simulink model "Solar_Vector_Control"  (R2024b)
settings: Solver=ode23t  StartTime=0.0  StopTime=2.5  RelTol=1e-3
libraries: spsCurrentMeasurementLib x6, spsVoltageMeasurementLib x4, spsSeriesRLCBranchLib x3, simulink x2, slpidlib x2, spsDiodeLib x1, spsIGBTLib x1, spsAsynchronousMachineSIUnitsLib x1, spsPVArrayLib x1, spsUniversalBridgeLib x1, spspowerguiLib x1
settings Model: Creator=ASUS  LastModifiedBy=ASUS
settings SolverCC: ZeroCrossControl=DisableAll

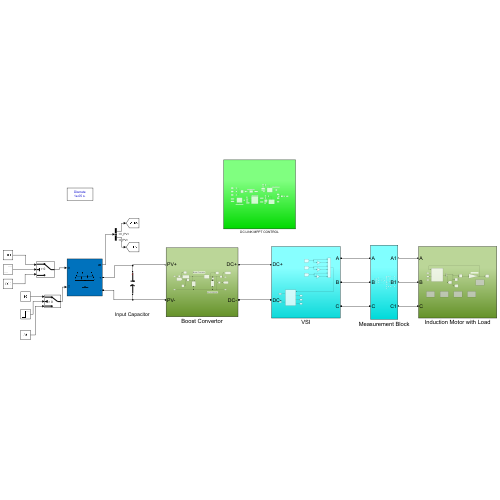
[thumbnail: Simulink's stored preview of the top-level diagram]
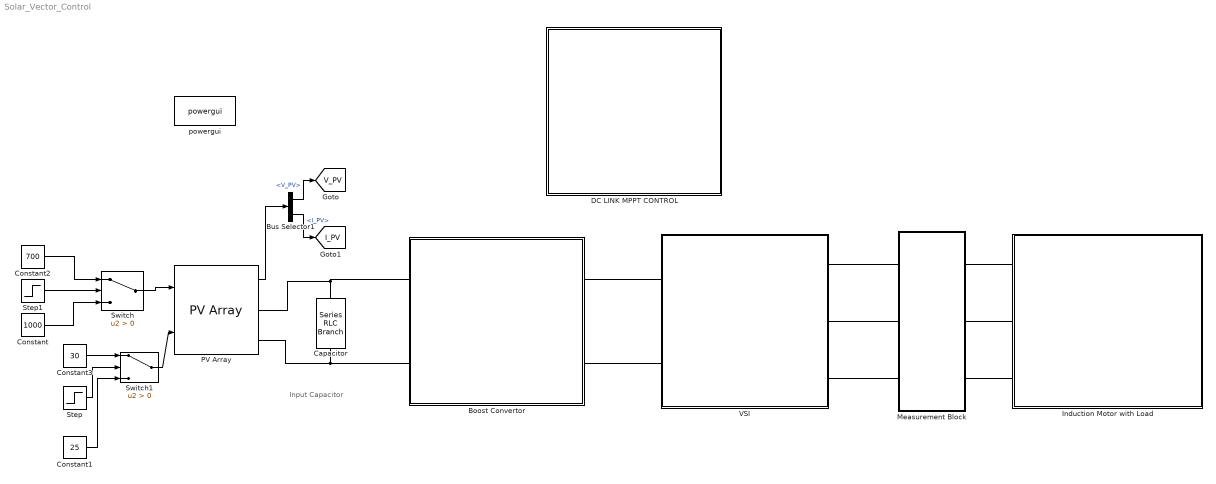
== system Solar_Vector_Control ==
  note: Input Capacitor
  Boost Convertor : Subsystem
  Bus Selector1 : BusSelector  OutputSignals=V_PV,I_PV
  Capacitor : spsSeriesRLCBranchLib/Series RLC Branch  LConnTagsString=__new0  RConnTagsString=__new0  BranchType=C  Resistance=1  Inductance=1e-3  SetiL0=off  InitialCurrent=0  Capacitance=100e-6  Setx0=off  InitialVoltage=0  Measurements=None
  Constant : Constant  Value=1000
  Constant1 : Constant  Value=25
  Constant2 : Constant  Value=700
  Constant3 : Constant  Value=30
  DC LINK MPPT CONTROL : Subsystem
  Induction Motor with Load : Subsystem
  Measurement Block : Subsystem
  PV Array : spsPVArrayLib/PV Array  Npar=2  Nser=12  PlotType=array @ 1000 W/m2 & specified temperatures  S_vec="[ 1000  500  100 ]"  Temp_C_vec="[ 45 25  ]"  ModuleName=User-defined  PlotWhenSelected=off  Pm=213.15  Ncell=60  Voc=36.3  Isc=7.84  Vm=29  Im=7.35  beta_Voc_pc=-0.36099  alpha_Isc_pc=0.102  beta_Voc=-0.13104  alpha_Isc=0.0079968  IL=7.8654  I0=2.9273e-10  nI=0.98119  Rsh=313.0553  Rs=0.39381  RobustModel=off  RobustCellTemperature=313.3991  BAL=on  Tc=1e-6  Tfilter=5e-5
  Step : Step  Time=5  SampleTime=0
  Step1 : Step  Time=3  SampleTime=0
  Switch : Switch  Criteria=u2 > Threshold  SaturateOnIntegerOverflow=off  InputSameDT=off
  Switch1 : Switch  Criteria=u2 > Threshold  SaturateOnIntegerOverflow=off  InputSameDT=off
  VSI : Subsystem
  powergui : spspowerguiLib/powergui  Priority=1  SimulationMode=Discrete  SampleTime=10e-6  frequency=60  Iterations=50  frequencyindice=0  Pbase=100e6  ErrMax=1e-4  UnitsV=kV  UnitsW=MW  buscounter=0  FunctionMessages=off  echomessages=off  EnableUseOfTLC=off  CurrentSourceSwitches=off  DisableSnubberDevices=off  DisableRonSwitches=off  DisableVfSwitches=off  DisplayEquations=off  AutomaticDiscreteSolvers=off  SolverType=Tustin/Backward Euler (TBE)  Interpol=off  ExternalGateDelay=off  methode=off  Ts=100  x0status=blocks  SPID=on  SwTol=0  HookPort=off  NonlinearTolerance=1e-4  nMaxIteration=100  ContinueOnMaxIteration=off  RestoreLinks=warning  ResistiveCurrentMeasurement=off  Frange=[0:2:500]  Ylog=off  Xlog=on  ShowGrid=off  save=off  variable=ZData  structure=0  ZoomFFT=off  StartTime=0.0  cycles=1  DisplayStyle=1  fundamental=60  FreqAxis=off  MaxFrequency=1000  frequencyindicesteady=1  RmsSteady=1  display=off
  tag scope: I_PV=global, V_PV=global
  wires:
  Switch/1 -> PV Array/1
  PV Array/1 -> Bus Selector1/1
  Bus Selector1/1 -> [V_PV]  "<V_PV>"
  Bus Selector1/2 -> [I_PV]  "<I_PV>"
  Constant/1 -> Switch/3
  Constant2/1 -> Switch/1
  Switch1/1 -> PV Array/2
  Constant1/1 -> Switch1/3
  Constant3/1 -> Switch1/1
  Step/1 -> Switch1/2
  Step1/1 -> Switch/2
  connections:
  PV Array/RConn1 -- Boost Convertor/LConn1 -- Capacitor/LConn1
  Capacitor/RConn1 -- PV Array/RConn2 -- Boost Convertor/LConn2
  Measurement Block/LConn1 -- VSI/LConn1
  VSI/LConn2 -- Measurement Block/LConn2
  Measurement Block/RConn2 -- Induction Motor with Load/LConn2
  Measurement Block/RConn1 -- Induction Motor with Load/LConn1
  Measurement Block/RConn3 -- Induction Motor with Load/LConn3
  Measurement Block/LConn3 -- VSI/LConn3
  Boost Convertor/RConn1 -- VSI/RConn1
  Boost Convertor/RConn2 -- VSI/RConn2

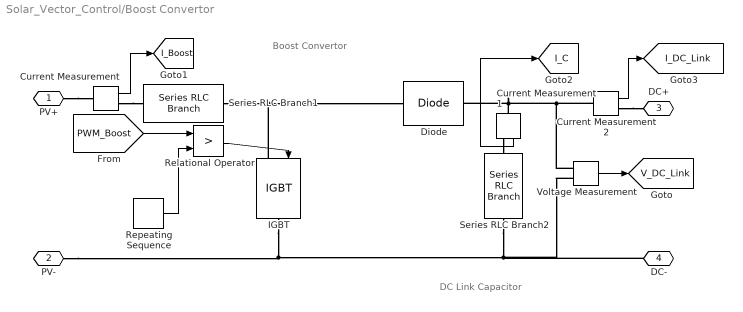
== system Solar_Vector_Control/Boost Convertor ==
  note: DC Link Capacitor
  note: Boost Convertor
  Current Measurement : spsCurrentMeasurementLib/Current Measurement  PhasorSimulation=off  OutputType=Complex  PSBequivalent=0
  Current Measurement1 : spsCurrentMeasurementLib/Current Measurement  PhasorSimulation=off  OutputType=Complex  PSBequivalent=0
  Current Measurement2 : spsCurrentMeasurementLib/Current Measurement  PhasorSimulation=off  OutputType=Complex  PSBequivalent=0
  Diode : spsDiodeLib/Diode  Ron=0.001  Lon=0  Vf=0.8  IC=0  UseSnubber=0  Rs=500  Cs=250e-9  Measurements=off
  IGBT : spsIGBTLib/IGBT  Ron=0.001  Lon=0  Vf=1  Tf=1e-6  Tt=2e-6  IC=0  Rs=1e5  Cs=inf  Measurements=off
  Relational Operator : RelationalOperator  Operator=>  OutDataTypeStr=boolean  RndMeth=Simplest  InputSameDT=off
  Repeating Sequence : simulink/Sources/Repeating Sequence  rep_seq_t=[0 25e-6 50e-6]  rep_seq_y=[0 1 0]
  Series RLC Branch1 : spsSeriesRLCBranchLib/Series RLC Branch  LConnTagsString=__new0  RConnTagsString=__new0  BranchType=L  Resistance=1  Inductance=3e-3  SetiL0=off  InitialCurrent=0  Capacitance=1e-6  Setx0=off  InitialVoltage=0  Measurements=None
  Series RLC Branch2 : spsSeriesRLCBranchLib/Series RLC Branch  LConnTagsString=__new0  RConnTagsString=__new0  BranchType=C  Resistance=1  Inductance=1e-3  SetiL0=off  InitialCurrent=0  Capacitance=1200e-6  Setx0=off  InitialVoltage=0  Measurements=None
  Voltage Measurement : spsVoltageMeasurementLib/Voltage Measurement  PhasorSimulation=off  OutputType=Complex  PSBequivalent=0
  PV+ : PMIOPort  Side=Left
  PV- : PMIOPort  Port=2  Side=Left
  DC+ : PMIOPort  Port=3  Side=Right
  DC- : PMIOPort  Port=4  Side=Right
  tag scope: I_Boost=global, I_C=global, I_DC_Link=global, V_DC_Link=global
  wires:
  Voltage Measurement/1 -> [V_DC_Link]
  [PWM_Boost] -> Relational Operator/1
  Repeating Sequence/1 -> Relational Operator/2
  Relational Operator/1 -> IGBT/1
  Current Measurement/1 -> [I_Boost]
  Current Measurement1/1 -> [I_C]
  Current Measurement2/1 -> [I_DC_Link]
  connections:
  Voltage Measurement/LConn1 -- Current Measurement1/LConn1 -- Diode/RConn1 -- Current Measurement2/LConn1
  IGBT/LConn1 -- Diode/LConn1 -- Series RLC Branch1/RConn1
  IGBT/RConn1 -- PV-/RConn1 -- Voltage Measurement/LConn2 -- DC-/RConn1 -- Series RLC Branch2/RConn1
  Current Measurement/RConn1 -- Series RLC Branch1/LConn1
  PV+/RConn1 -- Current Measurement/LConn1
  Current Measurement1/RConn1 -- Series RLC Branch2/LConn1
  Current Measurement2/RConn1 -- DC+/RConn1

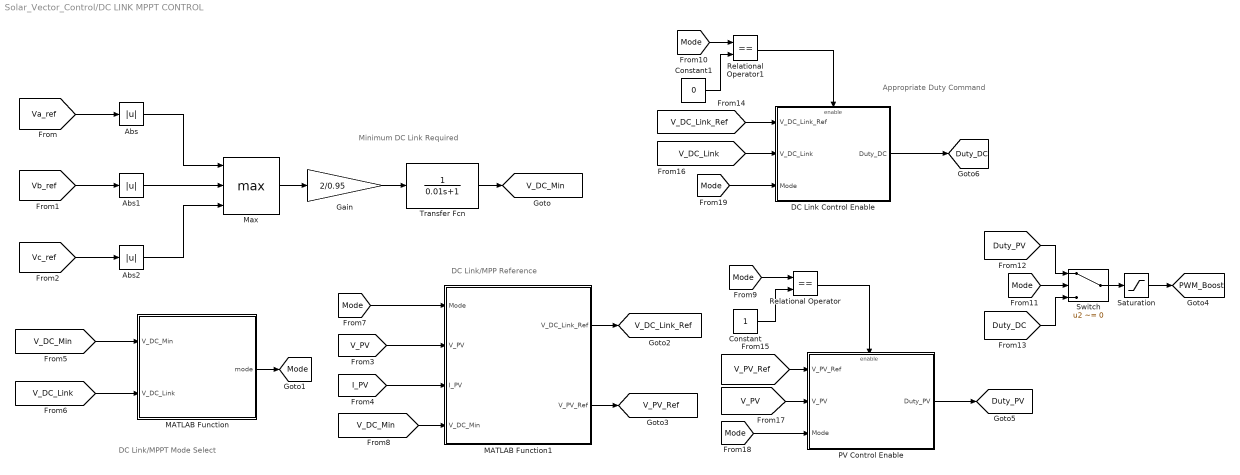
== system Solar_Vector_Control/DC LINK MPPT CONTROL ==
  note: Appropriate Duty Command
  note: DC Link/MPP Reference
  note: DC Link/MPPT Mode Select
  note: Minimum DC Link Required
  Abs : Abs  SaturateOnIntegerOverflow=off
  Abs1 : Abs  SaturateOnIntegerOverflow=off
  Abs2 : Abs  SaturateOnIntegerOverflow=off
  Constant : Constant
  Constant1 : Constant  Value=0
  DC Link Control Enable : Subsystem  TreatAsAtomicUnit=on
  Gain : Gain  Gain=2/0.95
  MATLAB Function : MATLAB Function  TreatAsAtomicUnit=on  SystemSampleTime=1e-5
  MATLAB Function1 : MATLAB Function  TreatAsAtomicUnit=on  SystemSampleTime=1e-5
  Max : MinMax  Function=max  Inputs=3
  PV Control Enable : Subsystem  TreatAsAtomicUnit=on
  Relational Operator : RelationalOperator  Operator===  OutDataTypeStr=boolean  RndMeth=Simplest  InputSameDT=off
  Relational Operator1 : RelationalOperator  Operator===  OutDataTypeStr=boolean  RndMeth=Simplest  InputSameDT=off
  Saturation : Saturate  UpperLimit=0.95  LowerLimit=0
  Switch : Switch  Criteria=u2 ~= 0  SaturateOnIntegerOverflow=off  InputSameDT=off
  Transfer Fcn : TransferFcn  Denominator=[0.01 1]
  tag scope: Duty_DC=global, Duty_PV=global, Mode=global, PWM_Boost=global, V_DC_Link_Ref=global, V_DC_Min=global, V_PV_Ref=global
  wires:
  [Va_ref] -> Abs/1
  [Vb_ref] -> Abs1/1
  [Vc_ref] -> Abs2/1
  Abs/1 -> Max/1
  Abs1/1 -> Max/2
  Abs2/1 -> Max/3
  Max/1 -> Gain/1
  [V_DC_Min] -> MATLAB Function/1(V_DC_Min)
  [V_DC_Link] -> MATLAB Function/2(V_DC_Link)
  MATLAB Function/1(mode) -> [Mode]
  [Mode] -> MATLAB Function1/1(Mode)
  [V_PV] -> MATLAB Function1/2(V_PV)
  [I_PV] -> MATLAB Function1/3(I_PV)
  [V_DC_Min] -> MATLAB Function1/4(V_DC_Min)
  MATLAB Function1/2(V_PV_Ref) -> [V_PV_Ref]
  Constant/1 -> Relational Operator/2
  [Mode] -> Relational Operator/1
  Relational Operator/1 -> PV Control Enable/Enable
  Relational Operator1/1 -> DC Link Control Enable/Enable
  Constant1/1 -> Relational Operator1/2
  [Mode] -> Relational Operator1/1
  [Mode] -> Switch/2
  [Duty_PV] -> Switch/1
  [Duty_DC] -> Switch/3
  Switch/1 -> Saturation/1
  Saturation/1 -> [PWM_Boost]
  [V_DC_Link_Ref] -> DC Link Control Enable/1(V_DC_Link_Ref)
  [V_PV_Ref] -> PV Control Enable/1(V_PV_Ref)
  [V_DC_Link] -> DC Link Control Enable/2(V_DC_Link)
  [V_PV] -> PV Control Enable/2(V_PV)
  PV Control Enable/1(Duty_PV) -> [Duty_PV]
  DC Link Control Enable/1(Duty_DC) -> [Duty_DC]
  [Mode] -> PV Control Enable/3(Mode)
  [Mode] -> DC Link Control Enable/3(Mode)
  Gain/1 -> Transfer Fcn/1
  Transfer Fcn/1 -> [V_DC_Min]
  MATLAB Function1/1(V_DC_Link_Ref) -> [V_DC_Link_Ref]

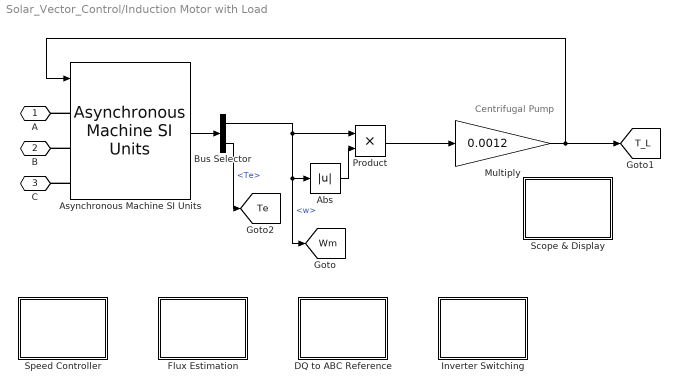
== system Solar_Vector_Control/Induction Motor with Load ==
  note: Centrifugal Pump
  Abs : Abs  SaturateOnIntegerOverflow=off
  Asynchronous Machine SI Units : spsAsynchronousMachineSIUnitsLib/Asynchronous Machine SI Units  RotorType=Squirrel-cage  PresetModel="15:  5.4 HP (4KW)   400 V  50Hz 1430 RPM"  MechanicalLoad=Torque Tm  ShowDetailedParameters=on  ReferenceFrame=Rotor  Units=SI  MeasurementBus=on  NominalParameters=[4000 400 50]  VoltageRatio=1  Stator=[1.405 0.005839]  Rotor=[1.395 0.005839]  Cage1=[0.4155 0.002066]  Cage2=[0.4168 0.0003495]  Lm=0.1722  Mechanical=[0.0131 0.002985 2]  PolePairs=2  InitialConditions=[1 0 0 0 0 0 0 0]  SimulateSaturation=off  Saturation=[14.03593122, 27.81365428, 53.79336849, 72.68890987, 97.98006896, 148.6815601, 215.7428561, 302.9841135, 428.7778367 ; 230, 322, 414, 460, 506, 552, 598, 644, 690]  LoadFlowParameters=1492000  TsPowergui=0  TsBlock=-1  IterativeModel=Trapezoidal non iterative  IterativeDiscreteModel=Trapezoidal non iterative  Pmec=1.492e+006
  Bus Selector : BusSelector  OutputSignals=w,Te
  DQ to ABC Reference : Subsystem
  Flux Estimation : Subsystem
  Inverter Switching : Subsystem
  Multiply : Gain  Gain=0.0012
  Product : Product
  Scope & Display : Subsystem
  Speed Controller : Subsystem
  A : PMIOPort  Side=Left
  B : PMIOPort  Port=2  Side=Left
  C : PMIOPort  Port=3  Side=Left
  tag scope: T_L=global, Te=global, Wm=global
  wires:
  Multiply/1 -> Asynchronous Machine SI Units/1, [T_L]
  Bus Selector/1 -> Product/1, Abs/1, [Wm]  "<w>"
  Asynchronous Machine SI Units/1 -> Bus Selector/1
  Product/1 -> Multiply/1
  Abs/1 -> Product/2
  Bus Selector/2 -> [Te]  "<Te>"
  connections:
  Asynchronous Machine SI Units/LConn1 -- A/RConn1
  Asynchronous Machine SI Units/LConn2 -- B/RConn1
  Asynchronous Machine SI Units/LConn3 -- C/RConn1

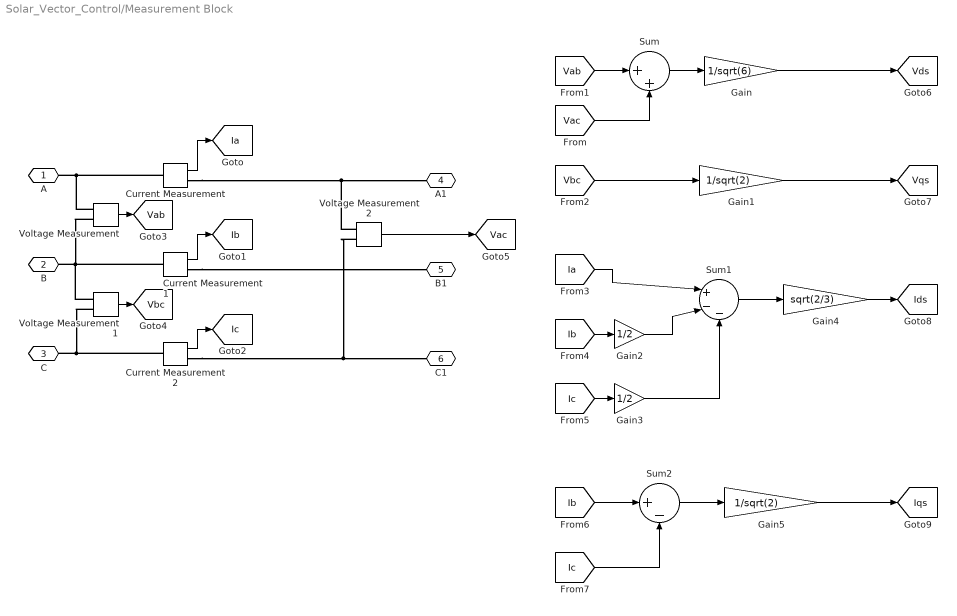
== system Solar_Vector_Control/Measurement Block ==
  Current Measurement : spsCurrentMeasurementLib/Current Measurement  PhasorSimulation=off  OutputType=Complex  PSBequivalent=0
  Current Measurement1 : spsCurrentMeasurementLib/Current Measurement  PhasorSimulation=off  OutputType=Complex  PSBequivalent=0
  Current Measurement2 : spsCurrentMeasurementLib/Current Measurement  PhasorSimulation=off  OutputType=Complex  PSBequivalent=0
  Gain : Gain  Gain=1/sqrt(6)
  Gain1 : Gain  Gain=1/sqrt(2)
  Gain2 : Gain  Gain=1/2
  Gain3 : Gain  Gain=1/2
  Gain4 : Gain  Gain=sqrt(2/3)
  Gain5 : Gain  Gain=1/sqrt(2)
  Sum : Sum  Inputs=|++
  Sum1 : Sum  Inputs=|+--
  Sum2 : Sum  Inputs=|+-
  Voltage Measurement : spsVoltageMeasurementLib/Voltage Measurement  PhasorSimulation=off  OutputType=Complex  PSBequivalent=0
  Voltage Measurement1 : spsVoltageMeasurementLib/Voltage Measurement  PhasorSimulation=off  OutputType=Complex  PSBequivalent=0
  Voltage Measurement2 : spsVoltageMeasurementLib/Voltage Measurement  PhasorSimulation=off  OutputType=Complex  PSBequivalent=0
  A : PMIOPort  Side=Left
  B : PMIOPort  Port=2  Side=Left
  C : PMIOPort  Port=3  Side=Left
  A1 : PMIOPort  Port=4  Side=Right
  B1 : PMIOPort  Port=5  Side=Right
  C1 : PMIOPort  Port=6  Side=Right
  tag scope: Ia=global, Ib=global, Ic=global, Ids=global, Iqs=global, Vab=global, Vac=global, Vbc=global, Vds=global, Vqs=global
  wires:
  Current Measurement/1 -> [Ia]
  Current Measurement1/1 -> [Ib]
  Current Measurement2/1 -> [Ic]
  Voltage Measurement/1 -> [Vab]
  Voltage Measurement1/1 -> [Vbc]
  Voltage Measurement2/1 -> [Vac]
  [Vab] -> Sum/1
  [Vac] -> Sum/2
  Sum/1 -> Gain/1
  Gain/1 -> [Vds]
  [Vbc] -> Gain1/1
  Gain1/1 -> [Vqs]
  [Ia] -> Sum1/1
  [Ib] -> Gain2/1
  Gain2/1 -> Sum1/2
  [Ic] -> Gain3/1
  Gain3/1 -> Sum1/3
  Sum1/1 -> Gain4/1
  Gain4/1 -> [Ids]
  [Ib] -> Sum2/1
  [Ic] -> Sum2/2
  Sum2/1 -> Gain5/1
  Gain5/1 -> [Iqs]
  connections:
  Current Measurement/LConn1 -- Voltage Measurement/LConn1 -- A/RConn1
  Current Measurement/RConn1 -- Voltage Measurement2/LConn1 -- A1/RConn1
  Current Measurement2/LConn1 -- Voltage Measurement1/LConn2 -- C/RConn1
  Current Measurement1/LConn1 -- Voltage Measurement1/LConn1 -- Voltage Measurement/LConn2 -- B/RConn1
  Current Measurement1/RConn1 -- B1/RConn1
  Current Measurement2/RConn1 -- Voltage Measurement2/LConn2 -- C1/RConn1

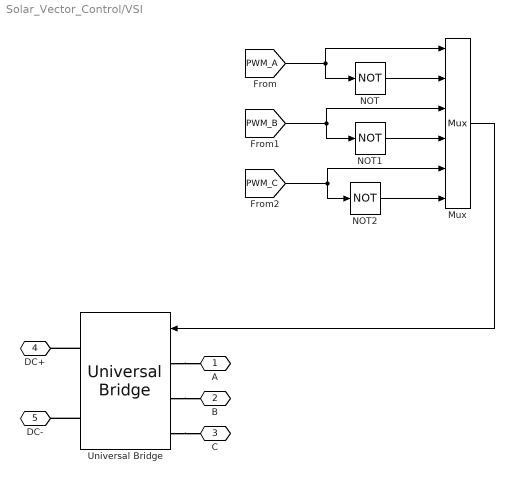
== system Solar_Vector_Control/VSI ==
  Mux : Mux  Inputs=6
  NOT : Logic  Operator=NOT  IconShape=distinctive  AllPortsSameDT=off  OutDataTypeStr=boolean
  NOT1 : Logic  Operator=NOT  IconShape=distinctive  AllPortsSameDT=off  OutDataTypeStr=boolean
  NOT2 : Logic  Operator=NOT  IconShape=distinctive  AllPortsSameDT=off  OutDataTypeStr=boolean
  Universal Bridge : spsUniversalBridgeLib/Universal Bridge  Arms=3  SnubberResistance=1e5  SnubberCapacitance=inf  Device=IGBT / Diodes  Ron=1e-3  Lon=0  ForwardVoltages="[  0  0  ]"  ForwardVoltage=0  GTOparameters=[ 10e-6 , 20e-6 ]  IGBTparameters=[ 1e-6 , 2e-6 ]  Measurements=None  Measurements_2=None  converterType=Rectifier
  A : PMIOPort  Side=Left
  B : PMIOPort  Port=2  Side=Left
  C : PMIOPort  Port=3  Side=Left
  DC+ : PMIOPort  Port=4  Side=Right
  DC- : PMIOPort  Port=5  Side=Right
  wires:
  NOT/1 -> Mux/2
  [PWM_A] -> Mux/1, NOT/1
  [PWM_B] -> Mux/3, NOT1/1
  [PWM_C] -> Mux/5, NOT2/1
  NOT2/1 -> Mux/6
  NOT1/1 -> Mux/4
  Mux/1 -> Universal Bridge/1
  connections:
  Universal Bridge/RConn2 -- DC-/RConn1
  Universal Bridge/LConn1 -- A/RConn1
  Universal Bridge/RConn1 -- DC+/RConn1
  Universal Bridge/LConn3 -- C/RConn1
  Universal Bridge/LConn2 -- B/RConn1

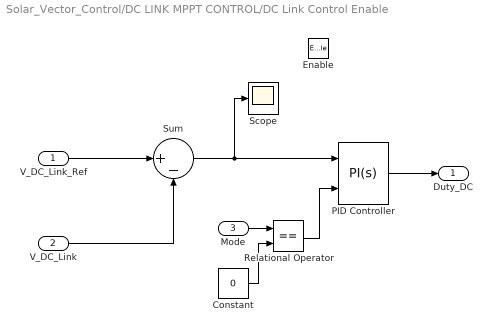
== system Solar_Vector_Control/DC LINK MPPT CONTROL/DC Link Control Enable ==
  V_DC_Link_Ref : Inport
  V_DC_Link : Inport  Port=2
  Mode : Inport  Port=3
  Enable : EnablePort
  Constant : Constant  Value=0
  PID Controller : slpidlib/PID Controller  Controller=PI  Form=Parallel  TimeDomain=Continuous-time  UseExternalTs=off  SampleTime=-1  IntegratorMethod=Forward Euler  FilterMethod=Forward Euler  ControllerParametersSource=internal  P=1e-6  I=0.04  UseKiTs=off  D=0  UseExternalDerivativeSource=off  N=100  UseFilter=on  TunerSelectOption=Transfer Function Based (PID Tuner App)  InitialConditionSource=internal  InitialConditionForIntegrator=0  InitialConditionForFilter=0  DifferentiatorICPrevScaledInput=0  ExternalReset=rising  TrackingMode=off  Kt=1  LimitOutput=on  SatLimitsSource=internal  UpperSaturationLimit=0.95  LowerSaturationLimit=0  LinearizeAsGain=on  AntiWindupMode=clamping  Kb=1  LimitIntegrator=off  UpperIntegratorSaturationLimit=inf  LowerIntegratorSaturationLimit=-inf  POutMin=[]  POutMax=[]  IOutMin=[]  IOutMax=[]  DOutMin=[]  DOutMax=[]  NOutMin=[]  NOutMax=[]  SumOutMin=[]  SumOutMax=[]  SaturationOutMin=[]  SaturationOutMax=[]  PParamMin=[]  PParamMax=[]  IParamMin=[]  IParamMax=[]  DParamMin=[]  DParamMax=[]  NParamMin=[]  NParamMax=[]  KbParamMin=[]  KbParamMax=[]  KtParamMin=[]  KtParamMax=[]  KbOutMin=[]  KbOutMax=[]  KtOutMin=[]  KtOutMax=[]  IntegratorOutMin=[]  IntegratorOutMax=[]  FilterOutMin=[]  FilterOutMax=[]  SumI1OutMin=[]  SumI1OutMax=[]  SumI2OutMin=[]  SumI2OutMax=[]  SumI3OutMin=[]  SumI3OutMax=[]  SumI4OutMin=[]  SumI4OutMax=[]  SumDOutMin=[]  SumDOutMax=[]  DifferentiatorOutMin=[]  DifferentiatorOutMax=[]  FilterDiffOutCoefMin=[]  FilterDiffOutCoefMax=[]  ReciprocalOutMin=[]  ReciprocalOutMax=[]  SumDenOutMin=[]  SumDenOutMax=[]  SumNumOutMin=[]  SumNumOutMax=[]  DivideOutMin=[]  DivideOutMax=[]  UdiffTsProdOutMin=[]  UdiffTsProdOutMax=[]  NTsProdOutMin=[]  NTsProdOutMax=[]  UintegralTsProdOutMin=[]  UintegralTsProdOutMax=[]  UngainTsProdOutMin=[]  UngainTsProdOutMax=[]  ClampingZeroOutDataTypeStr=Inherit: Inherit via back propagation  ClampingZeroOutMin=[]  ClampingZeroOutMax=[]  FilterDenConstantOutDataTypeStr=Inherit: Inherit via back propagation  FilterDenConstantOutMin=[]  FilterDenConstantOutMax=[]  PCopyOutDataTypeStr=Inherit: Inherit via back propagation  PCopyOutMin=[]  PCopyOutMax=[]  NCopyOutDataTypeStr=Inherit: Inherit via back propagation  NCopyOutMin=[]  NCopyOutMax=[]  IntegratorContinuousStateAttributes=''  IntegratorStateMustResolveToSignalObject=off  IntegratorRTWStateStorageClass=Auto  FilterContinuousStateAttributes=''  FilterStateMustResolveToSignalObject=off  FilterRTWStateStorageClass=Auto  ParallelPVariant=InternalParameters  IdealPVariant=Disabled  IVariant=InternalParameters  DVariant=Disabled  IntegratorVariant=Continuous  SatVariant=Enabled  AWVariant=ContClampingParallel  PCopyVariant=Disabled  TRVariant=Disabled  FdbkBlocksVariant=Forward  IdealPFdbkVariant=Disabled  SatFdbkVariant=Disabled  DerivativeFilterVariant=Disabled  NVariant=Disabled  NCopyVariant=Disabled_SignalSpec  FilterICVariant=Disabled  IntegratorICVariant=InternalICs  ExternalResetVariant=ExternalReset  TRSumVariant=Passthrough  SumFdbkVariant=Disabled  SumVariant=Sum_PI  TsampFilterVariant=InternalTs  TsampNgainVariant=Passthrough  TsampIntegralVariant=Disabled_SignalSpec  ExternalSaturationOutDataTypeStr=Inherit: Same as second input  DerivativeSourceVariant=Disabled  PreIntVariant=InternalPreInt
  Relational Operator : RelationalOperator  Operator===  OutDataTypeStr=boolean  RndMeth=Simplest  InputSameDT=off
  Scope : Scope
  Sum : Sum  Inputs=|+-
  Duty_DC : Outport
  wires:
  V_DC_Link_Ref/1 -> Sum/1
  V_DC_Link/1 -> Sum/2
  Sum/1 -> Scope/1, PID Controller/1
  PID Controller/1 -> Duty_DC/1
  Relational Operator/1 -> PID Controller/2
  Mode/1 -> Relational Operator/1
  Constant/1 -> Relational Operator/2

== system Solar_Vector_Control/DC LINK MPPT CONTROL/PV Control Enable ==
  V_PV_Ref : Inport
  V_PV : Inport  Port=2
  Mode : Inport  Port=3
  Enable : EnablePort
  Constant : Constant
  PID Controller : slpidlib/PID Controller  Controller=PI  Form=Parallel  TimeDomain=Continuous-time  UseExternalTs=off  SampleTime=-1  IntegratorMethod=Forward Euler  FilterMethod=Forward Euler  ControllerParametersSource=internal  P=1e-4  I=0.3  UseKiTs=off  D=0  UseExternalDerivativeSource=off  N=100  UseFilter=on  TunerSelectOption=Transfer Function Based (PID Tuner App)  InitialConditionSource=internal  InitialConditionForIntegrator=0  InitialConditionForFilter=0  DifferentiatorICPrevScaledInput=0  ExternalReset=rising  TrackingMode=off  Kt=1  LimitOutput=on  SatLimitsSource=internal  UpperSaturationLimit=0.95  LowerSaturationLimit=0  LinearizeAsGain=on  AntiWindupMode=clamping  Kb=1  LimitIntegrator=off  UpperIntegratorSaturationLimit=inf  LowerIntegratorSaturationLimit=-inf  POutMin=[]  POutMax=[]  IOutMin=[]  IOutMax=[]  DOutMin=[]  DOutMax=[]  NOutMin=[]  NOutMax=[]  SumOutMin=[]  SumOutMax=[]  SaturationOutMin=[]  SaturationOutMax=[]  PParamMin=[]  PParamMax=[]  IParamMin=[]  IParamMax=[]  DParamMin=[]  DParamMax=[]  NParamMin=[]  NParamMax=[]  KbParamMin=[]  KbParamMax=[]  KtParamMin=[]  KtParamMax=[]  KbOutMin=[]  KbOutMax=[]  KtOutMin=[]  KtOutMax=[]  IntegratorOutMin=[]  IntegratorOutMax=[]  FilterOutMin=[]  FilterOutMax=[]  SumI1OutMin=[]  SumI1OutMax=[]  SumI2OutMin=[]  SumI2OutMax=[]  SumI3OutMin=[]  SumI3OutMax=[]  SumI4OutMin=[]  SumI4OutMax=[]  SumDOutMin=[]  SumDOutMax=[]  DifferentiatorOutMin=[]  DifferentiatorOutMax=[]  FilterDiffOutCoefMin=[]  FilterDiffOutCoefMax=[]  ReciprocalOutMin=[]  ReciprocalOutMax=[]  SumDenOutMin=[]  SumDenOutMax=[]  SumNumOutMin=[]  SumNumOutMax=[]  DivideOutMin=[]  DivideOutMax=[]  UdiffTsProdOutMin=[]  UdiffTsProdOutMax=[]  NTsProdOutMin=[]  NTsProdOutMax=[]  UintegralTsProdOutMin=[]  UintegralTsProdOutMax=[]  UngainTsProdOutMin=[]  UngainTsProdOutMax=[]  ClampingZeroOutDataTypeStr=Inherit: Inherit via back propagation  ClampingZeroOutMin=[]  ClampingZeroOutMax=[]  FilterDenConstantOutDataTypeStr=Inherit: Inherit via back propagation  FilterDenConstantOutMin=[]  FilterDenConstantOutMax=[]  PCopyOutDataTypeStr=Inherit: Inherit via back propagation  PCopyOutMin=[]  PCopyOutMax=[]  NCopyOutDataTypeStr=Inherit: Inherit via back propagation  NCopyOutMin=[]  NCopyOutMax=[]  IntegratorContinuousStateAttributes=''  IntegratorStateMustResolveToSignalObject=off  IntegratorRTWStateStorageClass=Auto  FilterContinuousStateAttributes=''  FilterStateMustResolveToSignalObject=off  FilterRTWStateStorageClass=Auto  ParallelPVariant=InternalParameters  IdealPVariant=Disabled  IVariant=InternalParameters  DVariant=Disabled  IntegratorVariant=Continuous  SatVariant=Enabled  AWVariant=ContClampingParallel  PCopyVariant=Disabled  TRVariant=Disabled  FdbkBlocksVariant=Forward  IdealPFdbkVariant=Disabled  SatFdbkVariant=Disabled  DerivativeFilterVariant=Disabled  NVariant=Disabled  NCopyVariant=Disabled_SignalSpec  FilterICVariant=Disabled  IntegratorICVariant=InternalICs  ExternalResetVariant=ExternalReset  TRSumVariant=Passthrough  SumFdbkVariant=Disabled  SumVariant=Sum_PI  TsampFilterVariant=InternalTs  TsampNgainVariant=Passthrough  TsampIntegralVariant=Disabled_SignalSpec  ExternalSaturationOutDataTypeStr=Inherit: Same as second input  DerivativeSourceVariant=Disabled  PreIntVariant=InternalPreInt
  Relational Operator : RelationalOperator  Operator===  OutDataTypeStr=boolean  RndMeth=Simplest  InputSameDT=off
  Sum : Sum  Inputs=|-+
  Duty_PV : Outport
  wires:
  V_PV_Ref/1 -> Sum/1
  V_PV/1 -> Sum/2
  Sum/1 -> PID Controller/1
  PID Controller/1 -> Duty_PV/1
  Mode/1 -> Relational Operator/1
  Constant/1 -> Relational Operator/2
  Relational Operator/1 -> PID Controller/2

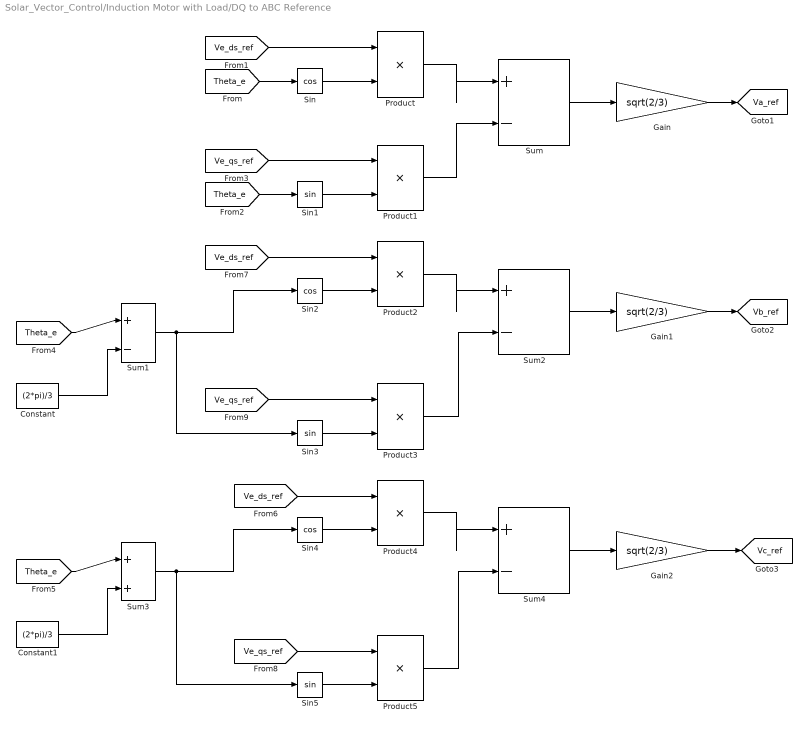
== system Solar_Vector_Control/Induction Motor with Load/DQ to ABC Reference ==
  Constant : Constant  Value=(2*pi)/3
  Constant1 : Constant  Value=(2*pi)/3
  Gain : Gain  Gain=sqrt(2/3)
  Gain1 : Gain  Gain=sqrt(2/3)
  Gain2 : Gain  Gain=sqrt(2/3)
  Product{,1..5} (6 alike) : Product
  Sin : Trigonometry  Operator=cos
  Sin1 : Trigonometry
  Sin2 : Trigonometry  Operator=cos
  Sin3 : Trigonometry
  Sin4 : Trigonometry  Operator=cos
  Sin5 : Trigonometry
  Sum{,1..2,4} (4 alike) : Sum  Inputs=|+-
  Sum3 : Sum  Inputs=|++
  tag scope: Va_ref=global, Vb_ref=global, Vc_ref=global
  wires:
  Sin/1 -> Product/2
  [Ve_ds_ref] -> Product/1
  Product/1 -> Sum/1
  [Theta_e] -> Sin1/1
  [Ve_qs_ref] -> Product1/1
  Sin1/1 -> Product1/2
  Product1/1 -> Sum/2
  Sum/1 -> Gain/1
  Gain/1 -> [Va_ref]
  [Ve_qs_ref] -> Product3/1
  Sum1/1 -> Sin2/1, Sin3/1
  [Ve_ds_ref] -> Product2/1
  Product3/1 -> Sum2/2
  Sin2/1 -> Product2/2
  Sum2/1 -> Gain1/1
  Sin3/1 -> Product3/2
  Product2/1 -> Sum2/1
  Gain1/1 -> [Vb_ref]
  Constant/1 -> Sum1/2
  Gain2/1 -> [Vc_ref]
  Product4/1 -> Sum4/1
  [Ve_qs_ref] -> Product5/1
  Sum4/1 -> Gain2/1
  [Theta_e] -> Sum3/1
  Sin5/1 -> Product5/2
  [Ve_ds_ref] -> Product4/1
  Constant1/1 -> Sum3/2
  Product5/1 -> Sum4/2
  Sum3/1 -> Sin4/1, Sin5/1
  Sin4/1 -> Product4/2
  [Theta_e] -> Sin/1
  [Theta_e] -> Sum1/1

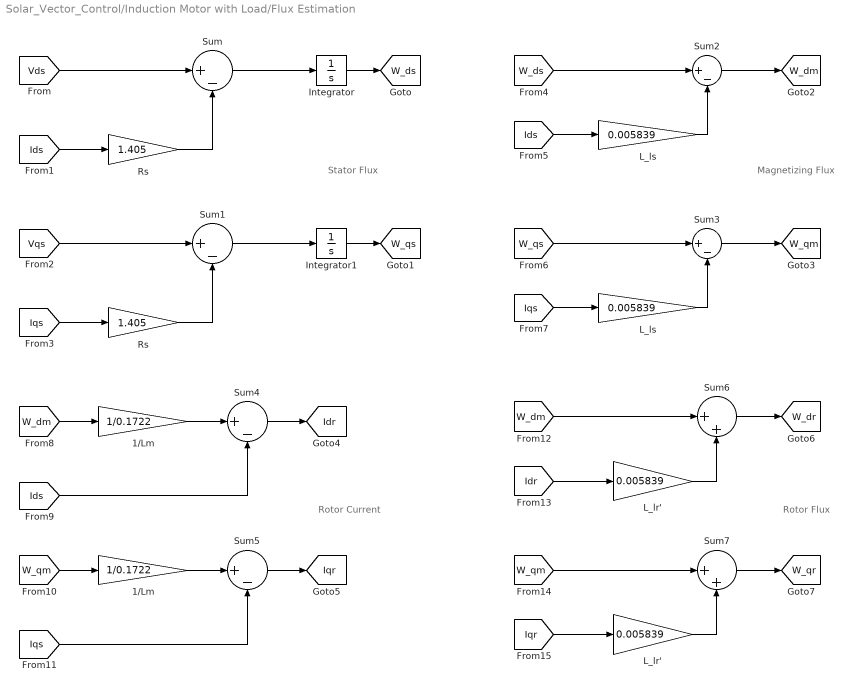
== system Solar_Vector_Control/Induction Motor with Load/Flux Estimation ==
  note: Rotor Flux
  note: Rotor Current
  note: Stator Flux
  note: Magnetizing Flux
  1/Lm : Gain  Gain=1/0.1722
  "1/Lm " : Gain  Gain=1/0.1722
  Integrator : Integrator
  Integrator1 : Integrator
  L_lr' : Gain  Gain=0.005839
  "L_lr' " : Gain  Gain=0.005839
  L_ls : Gain  Gain=0.005839
  "L_ls " : Gain  Gain=0.005839
  Rs : Gain  Gain=1.405
  "Rs " : Gain  Gain=1.405
  Sum{,1..5} (6 alike) : Sum  Inputs=|+-
  Sum6 : Sum  Inputs=|++
  Sum7 : Sum  Inputs=|++
  tag scope: Idr=global, Iqr=global, W_dm=global, W_dr=global, W_ds=global, W_qm=global, W_qr=global, W_qs=global
  wires:
  [Vds] -> Sum/1
  Rs/1 -> Sum/2
  Sum/1 -> Integrator/1
  [Ids] -> Rs/1
  Integrator/1 -> [W_ds]
  [Vqs] -> Sum1/1
  "Rs "/1 -> Sum1/2
  Integrator1/1 -> [W_qs]
  Sum1/1 -> Integrator1/1
  [Iqs] -> "Rs "/1
  [W_ds] -> Sum2/1
  [Ids] -> L_ls/1
  L_ls/1 -> Sum2/2
  [W_qs] -> Sum3/1
  [Iqs] -> "L_ls "/1
  "L_ls "/1 -> Sum3/2
  Sum2/1 -> [W_dm]
  Sum3/1 -> [W_qm]
  [W_dm] -> 1/Lm/1
  1/Lm/1 -> Sum4/1
  [Ids] -> Sum4/2
  Sum4/1 -> [Idr]
  Sum5/1 -> [Iqr]
  [Iqs] -> Sum5/2
  "1/Lm "/1 -> Sum5/1
  [W_qm] -> "1/Lm "/1
  [W_dm] -> Sum6/1
  [Idr] -> L_lr'/1
  L_lr'/1 -> Sum6/2
  Sum6/1 -> [W_dr]
  "L_lr' "/1 -> Sum7/2
  Sum7/1 -> [W_qr]
  [W_qm] -> Sum7/1
  [Iqr] -> "L_lr' "/1

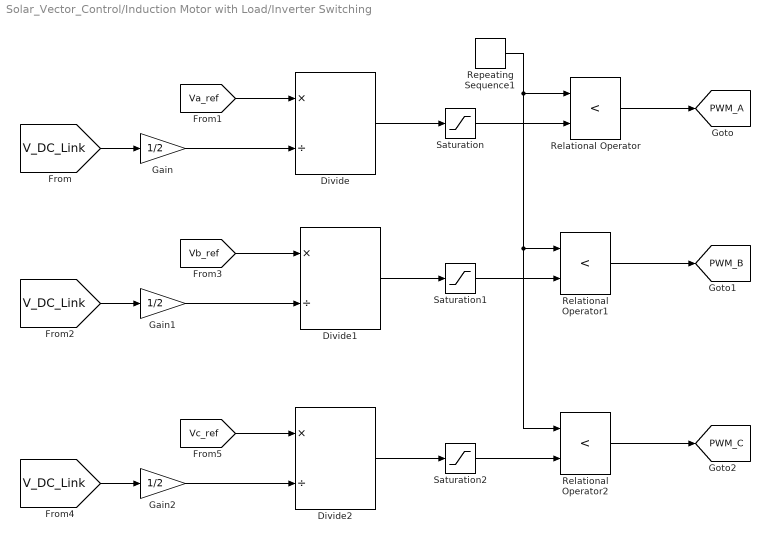
== system Solar_Vector_Control/Induction Motor with Load/Inverter Switching ==
  Divide : Product  Inputs=*/
  Divide1 : Product  Inputs=*/
  Divide2 : Product  Inputs=*/
  Gain : Gain  Gain=1/2
  Gain1 : Gain  Gain=1/2
  Gain2 : Gain  Gain=1/2
  Relational Operator : RelationalOperator  Operator=<  OutDataTypeStr=boolean  RndMeth=Simplest  InputSameDT=off
  Relational Operator1 : RelationalOperator  Operator=<  OutDataTypeStr=boolean  RndMeth=Simplest  InputSameDT=off
  Relational Operator2 : RelationalOperator  Operator=<  OutDataTypeStr=boolean  RndMeth=Simplest  InputSameDT=off
  Repeating Sequence1 : simulink/Sources/Repeating Sequence  rep_seq_t=[0 100e-6 200e-6]  rep_seq_y=[-1 1 -1]
  Saturation : Saturate  UpperLimit=1  LowerLimit=-1
  Saturation1 : Saturate  UpperLimit=1  LowerLimit=-1
  Saturation2 : Saturate  UpperLimit=1  LowerLimit=-1
  tag scope: PWM_A=global, PWM_B=global, PWM_C=global
  wires:
  Divide/1 -> Saturation/1
  Gain/1 -> Divide/2
  [V_DC_Link] -> Gain/1
  [Va_ref] -> Divide/1
  [V_DC_Link] -> Gain1/1
  Gain1/1 -> Divide1/2
  [Vb_ref] -> Divide1/1
  Divide1/1 -> Saturation1/1
  [V_DC_Link] -> Gain2/1
  Gain2/1 -> Divide2/2
  [Vc_ref] -> Divide2/1
  Divide2/1 -> Saturation2/1
  Saturation/1 -> Relational Operator/2
  Saturation1/1 -> Relational Operator1/2
  Saturation2/1 -> Relational Operator2/2
  Relational Operator2/1 -> [PWM_C]
  Relational Operator1/1 -> [PWM_B]
  Relational Operator/1 -> [PWM_A]
  Repeating Sequence1/1 -> Relational Operator2/1, Relational Operator1/1, Relational Operator/1

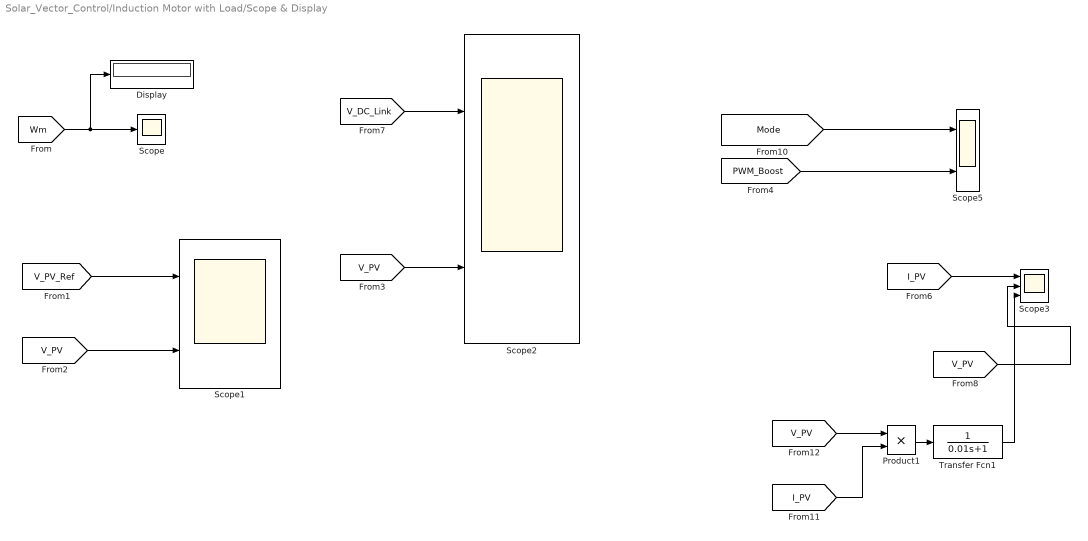
== system Solar_Vector_Control/Induction Motor with Load/Scope & Display ==
  Display : Display
  Product1 : Product
  Scope : Scope
  Scope1 : Scope  NumInputPorts=2
  Scope2 : Scope  NumInputPorts=2
  Scope3 : Scope  NumInputPorts=3
  Scope5 : Scope  NumInputPorts=2
  Transfer Fcn1 : TransferFcn  Denominator=[0.01 1]
  wires:
  [Wm] -> Display/1, Scope/1
  [V_PV_Ref] -> Scope1/1
  [V_PV] -> Scope3/2
  [V_DC_Link] -> Scope2/1
  [V_PV] -> Product1/1
  [PWM_Boost] -> Scope5/2
  Transfer Fcn1/1 -> Scope3/3
  [I_PV] -> Scope3/1
  [I_PV] -> Product1/2
  Product1/1 -> Transfer Fcn1/1
  [Mode] -> Scope5/1
  [V_PV] -> Scope1/2
  [V_PV] -> Scope2/2

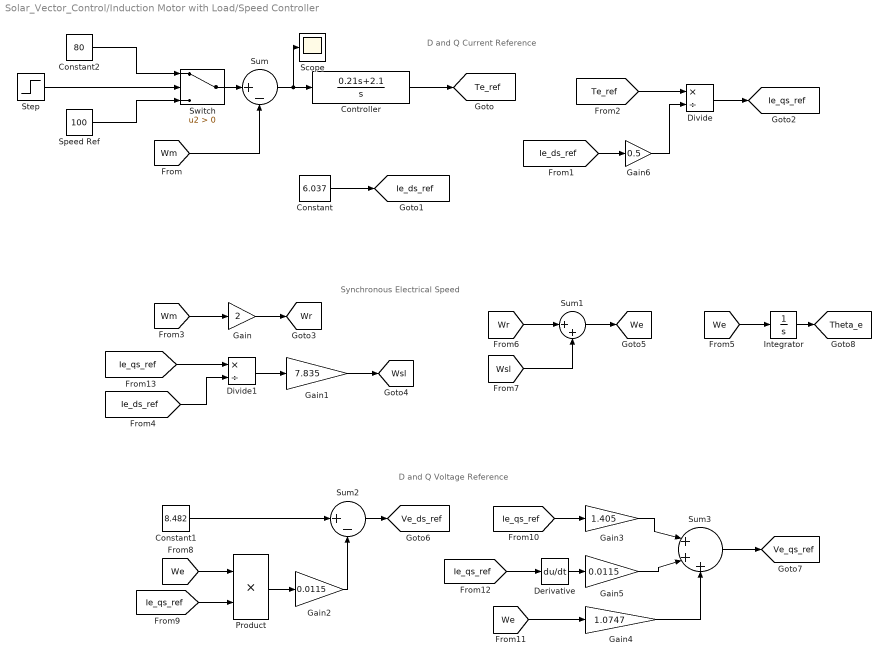
== system Solar_Vector_Control/Induction Motor with Load/Speed Controller ==
  note: D and Q Voltage Reference
  note: Synchronous Electrical Speed
  note: D and Q Current Reference
  Constant : Constant  Value=6.037
  Constant1 : Constant  Value=8.482
  Constant2 : Constant  Value=80
  Controller : TransferFcn  Numerator=[0.21 2.1]  Denominator=[1 0]
  Derivative : Derivative
  Divide : Product  Inputs=*/
  Divide1 : Product  Inputs=*/
  Gain : Gain  Gain=2
  Gain1 : Gain  Gain=7.835
  Gain2 : Gain  Gain=0.0115
  Gain3 : Gain  Gain=1.405
  Gain4 : Gain  Gain=1.0747
  Gain5 : Gain  Gain=0.0115
  Gain6 : Gain  Gain=0.5
  Integrator : Integrator
  Product : Product
  Scope : Scope
  Speed Ref : Constant  Value=100
  Step : Step  Time=7  SampleTime=0
  Sum : Sum  Inputs=|+-
  Sum1 : Sum  Inputs=|++
  Sum2 : Sum  Inputs=|+-
  Sum3 : Sum  Inputs=|+++
  Switch : Switch  Criteria=u2 > Threshold  SaturateOnIntegerOverflow=off  InputSameDT=off
  tag scope: Ie_ds_ref=global, Ie_qs_ref=global, Te_ref=global, Theta_e=global, Ve_ds_ref=global, Ve_qs_ref=global, We=global, Wr=global, Wsl=global
  wires:
  [Wm] -> Sum/2
  Sum/1 -> Scope/1, Controller/1
  Controller/1 -> [Te_ref]
  Constant/1 -> [Ie_ds_ref]
  [Te_ref] -> Divide/1
  Divide/1 -> [Ie_qs_ref]
  [Wm] -> Gain/1
  Gain/1 -> [Wr]
  [Ie_qs_ref] -> Divide1/1
  Divide1/1 -> Gain1/1
  Gain1/1 -> [Wsl]
  [Wr] -> Sum1/1
  [Wsl] -> Sum1/2
  Constant1/1 -> Sum2/1
  [We] -> Product/1
  [Ie_qs_ref] -> Product/2
  Sum2/1 -> [Ve_ds_ref]
  Gain2/1 -> Sum2/2
  Product/1 -> Gain2/1
  [Ie_qs_ref] -> Gain3/1
  Gain3/1 -> Sum3/1
  [We] -> Gain4/1
  Gain4/1 -> Sum3/3
  Derivative/1 -> Gain5/1
  [Ie_qs_ref] -> Derivative/1
  Gain5/1 -> Sum3/2
  Sum3/1 -> [Ve_qs_ref]
  Sum1/1 -> [We]
  [Ie_ds_ref] -> Divide1/2
  [We] -> Integrator/1
  Integrator/1 -> [Theta_e]
  [Ie_ds_ref] -> Gain6/1
  Gain6/1 -> Divide/2
  Switch/1 -> Sum/1
  Speed Ref/1 -> Switch/3
  Constant2/1 -> Switch/1
  Step/1 -> Switch/2

== matlab function Solar_Vector_Control/DC LINK MPPT CONTROL/MATLAB Function1 ==
  data: V_DC_Link_Ref output; Mode input; V_PV input; I_PV input; V_DC_Min input; V_PV_Ref output
function [V_DC_Link_Ref,V_PV_Ref] = fcn(Mode,V_PV,I_PV,V_DC_Min)

%MPPT Parameters
Vref_Max  = 430;
Vref_Min  = 200;
Vref_Init = 348;
DeltaVref = 1;

%Memory
persistent V_PV_Old I_PV_Old V_PV_Ref_Old

if isempty(V_PV_Old)

    V_PV_Old     = V_PV;
    I_PV_Old     = I_PV;
    V_PV_Ref_Old = Vref_Init;

end

% Default outputs
V_DC_Link_Ref = 0;
V_PV_Ref      = 0;

% MODE 0
% DC-Link Regulation

if Mode == 0

    V_DC_Link_Ref = V_DC_Min;

% MODE 1
% Incremental Conductance MPPT

else

    dV = V_PV - V_PV_Old;
    dI = I_PV - I_PV_Old;

    if abs(dV) < 1e-6

        if abs(dI) < 1e-6

            V_PV_Ref = V_PV_Ref_Old;

        elseif dI > 0

            V_PV_Ref = V_PV_Ref_Old + DeltaVref;

        else

            V_PV_Ref = V_PV_Ref_Old - DeltaVref;

        end

    else

        IncCond  = dI/dV;
        InstCond = -I_PV/V_PV;

        if abs(IncCond-InstCond) < 1e-6

            V_PV_Ref = V_PV_Ref_Old;

        elseif IncCond > InstCond

            V_PV_Ref = V_PV_Ref_Old + DeltaVref;

        else

            V_PV_Ref = V_PV_Ref_Old - DeltaVref;

        end

    end

    % Voltage Limits
    if V_PV_Ref > Vref_Max

        V_PV_Ref = Vref_Max;

    elseif V_PV_Ref < Vref_Min

        V_PV_Ref = Vref_Min;

    end

    % Update Memory
    V_PV_Old = V_PV;
    I_PV_Old = I_PV;
    V_PV_Ref_Old = V_PV_Ref;

end

end

== matlab function Solar_Vector_Control/DC LINK MPPT CONTROL/MATLAB Function ==
  data: V_DC_Min input; mode output; V_DC_Link input
function mode = fcn(V_DC_Min, V_DC_Link)

persistent mode_state

if isempty(mode_state)
    mode_state = 0;      % Start in DC-Link mode
end

H = 0.02;

if mode_state == 0

    if V_DC_Link > (1 + H)*V_DC_Min
        mode_state = 1; % Switch to MPPT
    end

else

    if V_DC_Link < V_DC_Min
        mode_state = 0; % Switch to DC-Link
    end

end

% Output
mode = mode_state;

end
